simulink model "PIDController_theta2"  (R2022a)
settings: Solver=ode5  StartTime=0.0  StopTime=2.4478  FixedStep=0.061194  RelTol=1e-3
settings Model: Creator=Admin  LastModifiedBy=mquyet
settings SolverCC: AlgebraicLoopSolver=TrustRegion
settings DataIOCC: ReturnWorkspaceOutputs=off
settings DebuggingCC: UnconnectedInputMsg=warning  UnconnectedOutputMsg=warning  UnconnectedLineMsg=warning  SFMachineParentedDataDiag=warning  ArithmeticOperatorsInVariantConditions=warning
settings SFSimCC: SimUseLocalCustomCode=off  CustomCodeUndefinedFunction=UseInterfaceOnly
settings RTWCC: RTWUseLocalCustomCode=off
settings CodeAppCC: StateflowObjectComments=on

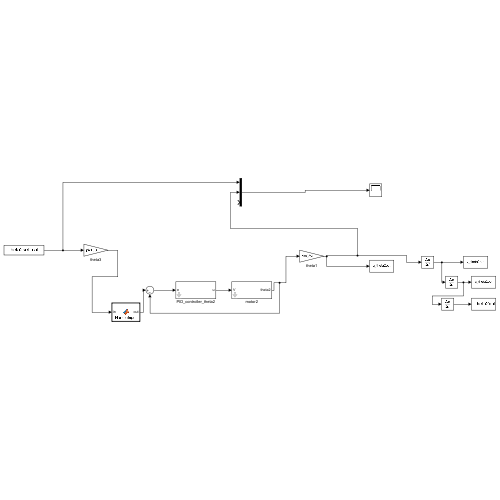
[thumbnail: Simulink's stored preview of the top-level diagram]
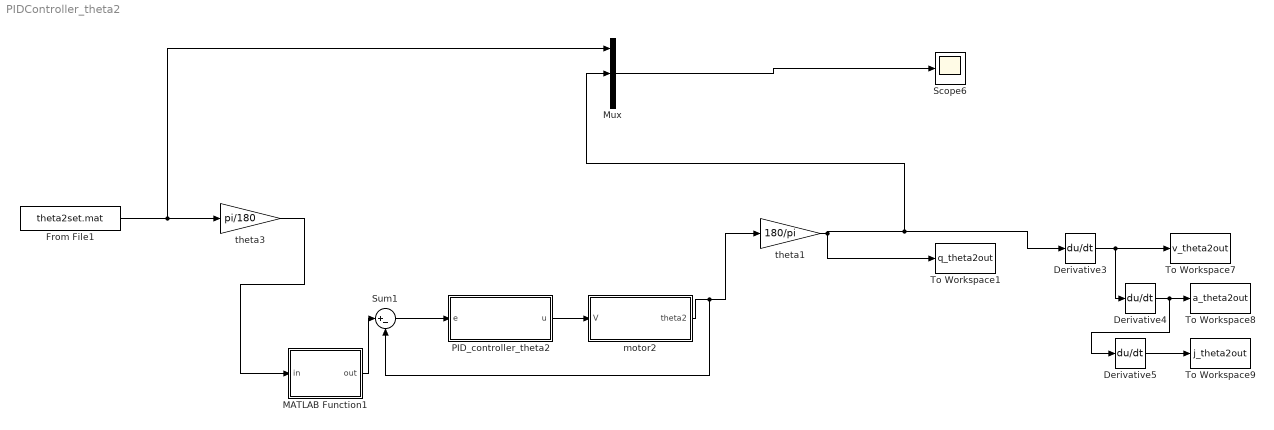
== system PIDController_theta2 ==
  Derivative3 : Derivative
  Derivative4 : Derivative
  Derivative5 : Derivative
  From File1 : FromFile  FileName=theta2set.mat
  MATLAB Function1 : MATLAB Function  TreatAsAtomicUnit=on
  Mux : Mux  Inputs=3
  PID_controller_theta2 : Subsystem  mask{Kp=10000, Ki=0, Kd=0}
  Scope6 : Scope
  Sum1 : Sum  Inputs=|+-
  To Workspace1 : ToWorkspace  VariableName=q_theta2out  SampleTime=-1
  To Workspace7 : ToWorkspace  VariableName=v_theta2out  SampleTime=-1
  To Workspace8 : ToWorkspace  VariableName=a_theta2out  SampleTime=-1
  To Workspace9 : ToWorkspace  VariableName=j_theta2out  SampleTime=-1
  motor2 : Subsystem  mask{Ki=0.1, Kb=0.1, L=0.5, R=2, Jeff=0.02, Beff=0.2, N=100}
  theta1 : Gain  Gain=180/pi
  theta3 : Gain  Gain=pi/180
  wires:
  Derivative3/1 -> Derivative4/1, To Workspace7/1
  Derivative4/1 -> Derivative5/1, To Workspace8/1
  Derivative5/1 -> To Workspace9/1
  theta1/1 -> Mux/2, Derivative3/1, To Workspace1/1
  From File1/1 -> Mux/1, theta3/1
  Mux/1 -> Scope6/1
  motor2/1(theta2) -> Sum1/2, theta1/1
  MATLAB Function1/1(out) -> Sum1/1
  theta3/1 -> MATLAB Function1/1(in)
  Sum1/1 -> PID_controller_theta2/1(e)
  PID_controller_theta2/1(u) -> motor2/1(V)

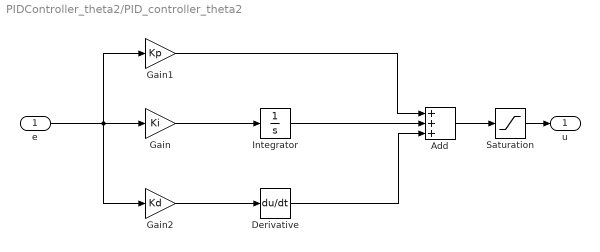
== system PIDController_theta2/PID_controller_theta2 ==
  e : Inport
  Add : Sum  Inputs=+++
  Derivative : Derivative
  Gain : Gain  Gain=Ki
  Gain1 : Gain  Gain=Kp
  Gain2 : Gain  Gain=Kd
  Integrator : Integrator
  Saturation : Saturate  UpperLimit=300  LowerLimit=-300
  u : Outport  VectorParamsAs1DForOutWhenUnconnected=off
  wires:
  e/1 -> Gain2/1, Gain1/1, Gain/1
  Gain/1 -> Integrator/1
  Gain2/1 -> Derivative/1
  Gain1/1 -> Add/1
  Integrator/1 -> Add/2
  Derivative/1 -> Add/3
  Add/1 -> Saturation/1
  Saturation/1 -> u/1

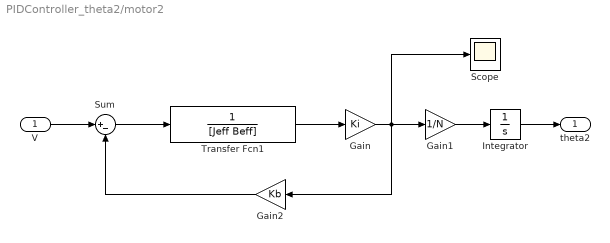
== system PIDController_theta2/motor2 ==
  V : Inport
  Gain : Gain  Gain=Ki
  Gain1 : Gain  Gain=1/N
  Gain2 : Gain  Gain=Kb
  Integrator : Integrator  InitialCondition=90
  Scope : Scope
  Sum : Sum  Inputs=|+-
  Transfer Fcn1 : TransferFcn  Denominator=[Jeff Beff]
  theta2 : Outport  VectorParamsAs1DForOutWhenUnconnected=off
  wires:
  Transfer Fcn1/1 -> Gain/1
  Gain1/1 -> Integrator/1
  Gain2/1 -> Sum/2
  V/1 -> Sum/1
  Sum/1 -> Transfer Fcn1/1
  Gain/1 -> Gain1/1, Gain2/1, Scope/1
  Integrator/1 -> theta2/1

== matlab function PIDController_theta2/MATLAB Function1 ==
  settings: updateMethod=DISCRETE
  data: in input; out output
function out = HandleInput(in)

out = in
persistent pre
if isempty(pre)
    pre = 0;
end

while (out - pre > 1.5*pi)
    out = out - 2*pi;
end

while (out - pre < -1.5*pi)
    out = out + 2*pi;
end
